simulink model "Quad_Nonlinear_Pitch_OL"  (R2020a)
settings: Solver=ode4  StartTime=0.0  StopTime=0.4  FixedStep=0.02  RelTol=1e-3
values from neighbouring files (symbols this model uses):
  B1 = (h_cg * g * m_tot) / (m_tot * h_cg^2 + J_yy)    [QuadConstants.m]    (also in pitch_parameter_estiation_result.m = 4.3602681386)
  B3 = (b * d_cg) / (m_tot * h_cg^2 + J_yy)    [QuadConstants.m]    (also in pitch_parameter_estiation_result.m = 7.12739951624e-05)
  B5 = (m2 * g * miu_k * r_y) / (m_tot * h_cg^2 + J_yy)    [QuadConstants.m]    (also in pitch_parameter_estiation_result.m = 0.59598011023)
  B6 = 2    [QuadConstants.m]    (also in pitch_parameter_estiation_result.m = 4.42876359313)
  init_I = data_I(1, :)    [load_data.m]
  init_II = data_II(1, :)    [load_data.m]
  init_III = data_III(1, :)    [load_data.m]
  init_IV = data_IV(1, :)    [load_data.m]
  init_V = data_V(1, :)    [load_data.m]
undefined symbols (not defined in the file or in its folder): magnitude
settings Model: OrderedModelArguments=off  Creator=Ali  LastModifiedBy=Ali

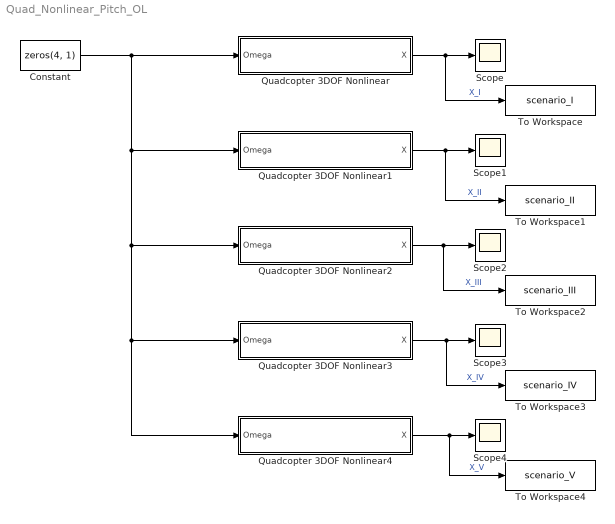
== system Quad_Nonlinear_Pitch_OL ==
  Constant : Constant  Value=zeros(4, 1)
  Quadcopter 3DOF Nonlinear : Subsystem  TreatAsAtomicUnit=on
  Quadcopter 3DOF Nonlinear1 : Subsystem  TreatAsAtomicUnit=on
  Quadcopter 3DOF Nonlinear2 : Subsystem  TreatAsAtomicUnit=on
  Quadcopter 3DOF Nonlinear3 : Subsystem  TreatAsAtomicUnit=on
  Quadcopter 3DOF Nonlinear4 : Subsystem  TreatAsAtomicUnit=on
  Scope{,1..4} (5 alike) : Scope
  To Workspace : ToWorkspace  VariableName=scenario_I  SampleTime=-1
  To Workspace1 : ToWorkspace  VariableName=scenario_II  SampleTime=-1
  To Workspace2 : ToWorkspace  VariableName=scenario_III  SampleTime=-1
  To Workspace3 : ToWorkspace  VariableName=scenario_IV  SampleTime=-1
  To Workspace4 : ToWorkspace  VariableName=scenario_V  SampleTime=-1
  wires:
  Quadcopter 3DOF Nonlinear/1(X) -> To Workspace/1, Scope/1  "X_I"
  Quadcopter 3DOF Nonlinear1/1(X) -> To Workspace1/1, Scope1/1  "X_II"
  Quadcopter 3DOF Nonlinear2/1(X) -> To Workspace2/1, Scope2/1  "X_III"
  Quadcopter 3DOF Nonlinear3/1(X) -> To Workspace3/1, Scope3/1  "X_IV"
  Quadcopter 3DOF Nonlinear4/1(X) -> To Workspace4/1, Scope4/1  "X_V"
  Constant/1 -> Quadcopter 3DOF Nonlinear4/1(Omega), Quadcopter 3DOF Nonlinear3/1(Omega), Quadcopter 3DOF Nonlinear2/1(Omega), Quadcopter 3DOF Nonlinear1/1(Omega), Quadcopter 3DOF Nonlinear/1(Omega)

== system Quad_Nonlinear_Pitch_OL/Quadcopter 3DOF Nonlinear ==
  Omega : Inport
  Integrator : Integrator  InitialCondition=init_I
  Quad System : Subsystem
  X : Outport
  wires:
  Integrator/1 -> Quad System/1(X), X/1  "X"
  Quad System/1(dot(X)) -> Integrator/1  "dot(X)"
  Omega/1 -> Quad System/2(Omega)

== system Quad_Nonlinear_Pitch_OL/Quadcopter 3DOF Nonlinear1 ==
  Omega : Inport
  Integrator : Integrator  InitialCondition=init_II
  Quad System : Subsystem
  X : Outport
  wires:
  Integrator/1 -> Quad System/1(X), X/1  "X"
  Quad System/1(dot(X)) -> Integrator/1  "dot(X)"
  Omega/1 -> Quad System/2(Omega)

== system Quad_Nonlinear_Pitch_OL/Quadcopter 3DOF Nonlinear2 ==
  Omega : Inport
  Integrator : Integrator  InitialCondition=init_III
  Quad System : Subsystem
  X : Outport
  wires:
  Integrator/1 -> Quad System/1(X), X/1  "X"
  Quad System/1(dot(X)) -> Integrator/1  "dot(X)"
  Omega/1 -> Quad System/2(Omega)

== system Quad_Nonlinear_Pitch_OL/Quadcopter 3DOF Nonlinear3 ==
  Omega : Inport
  Integrator : Integrator  InitialCondition=init_IV
  Quad System : Subsystem
  X : Outport
  wires:
  Integrator/1 -> Quad System/1(X), X/1  "X"
  Quad System/1(dot(X)) -> Integrator/1  "dot(X)"
  Omega/1 -> Quad System/2(Omega)

== system Quad_Nonlinear_Pitch_OL/Quadcopter 3DOF Nonlinear4 ==
  Omega : Inport
  Integrator : Integrator  InitialCondition=init_V
  Quad System : Subsystem
  X : Outport
  wires:
  Integrator/1 -> Quad System/1(X), X/1  "X"
  Quad System/1(dot(X)) -> Integrator/1  "dot(X)"
  Omega/1 -> Quad System/2(Omega)

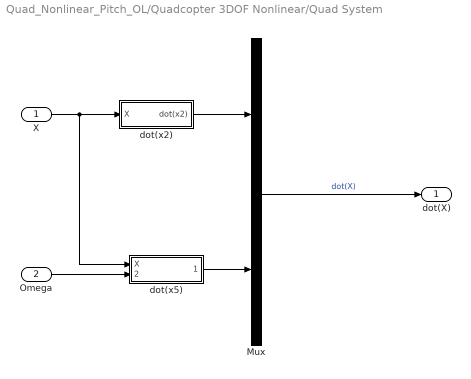
== system Quad_Nonlinear_Pitch_OL/Quadcopter 3DOF Nonlinear/Quad System ==
  X : Inport
  Omega : Inport  Port=2
  Mux : Mux  Inputs=2
  dot(x2) : Subsystem
  dot(x5) : Subsystem
  dot(X) : Outport
  wires:
  Mux/1 -> dot(X)/1  "dot(X)"
  dot(x2)/1(dot(x2)) -> Mux/1
  dot(x5)/1(dot(x5)) -> Mux/2
  X/1 -> dot(x5)/1(X), dot(x2)/1(X)
  Omega/1 -> dot(x5)/2(Omega)

== system Quad_Nonlinear_Pitch_OL/Quadcopter 3DOF Nonlinear1/Quad System ==
  X : Inport
  Omega : Inport  Port=2
  Mux : Mux  Inputs=2
  dot(x2) : Subsystem
  dot(x5) : Subsystem
  dot(X) : Outport
  wires:
  Mux/1 -> dot(X)/1  "dot(X)"
  dot(x2)/1(dot(x2)) -> Mux/1
  dot(x5)/1(dot(x5)) -> Mux/2
  X/1 -> dot(x5)/1(X), dot(x2)/1(X)
  Omega/1 -> dot(x5)/2(Omega)

== system Quad_Nonlinear_Pitch_OL/Quadcopter 3DOF Nonlinear2/Quad System ==
  X : Inport
  Omega : Inport  Port=2
  Mux : Mux  Inputs=2
  dot(x2) : Subsystem
  dot(x5) : Subsystem
  dot(X) : Outport
  wires:
  Mux/1 -> dot(X)/1  "dot(X)"
  dot(x2)/1(dot(x2)) -> Mux/1
  dot(x5)/1(dot(x5)) -> Mux/2
  X/1 -> dot(x5)/1(X), dot(x2)/1(X)
  Omega/1 -> dot(x5)/2(Omega)

== system Quad_Nonlinear_Pitch_OL/Quadcopter 3DOF Nonlinear3/Quad System ==
  X : Inport
  Omega : Inport  Port=2
  Mux : Mux  Inputs=2
  dot(x2) : Subsystem
  dot(x5) : Subsystem
  dot(X) : Outport
  wires:
  Mux/1 -> dot(X)/1  "dot(X)"
  dot(x2)/1(dot(x2)) -> Mux/1
  dot(x5)/1(dot(x5)) -> Mux/2
  X/1 -> dot(x5)/1(X), dot(x2)/1(X)
  Omega/1 -> dot(x5)/2(Omega)

== system Quad_Nonlinear_Pitch_OL/Quadcopter 3DOF Nonlinear4/Quad System ==
  X : Inport
  Omega : Inport  Port=2
  Mux : Mux  Inputs=2
  dot(x2) : Subsystem
  dot(x5) : Subsystem
  dot(X) : Outport
  wires:
  Mux/1 -> dot(X)/1  "dot(X)"
  dot(x2)/1(dot(x2)) -> Mux/1
  dot(x5)/1(dot(x5)) -> Mux/2
  X/1 -> dot(x5)/1(X), dot(x2)/1(X)
  Omega/1 -> dot(x5)/2(Omega)

== system Quad_Nonlinear_Pitch_OL/Quadcopter 3DOF Nonlinear/Quad System/dot(x2) ==
  X : Inport
  1 : Subsystem
  dot(x2) : Outport
  wires:
  X/1 -> 1/1(X)  "X"
  1/1(x5cos(x1)) -> dot(x2)/1

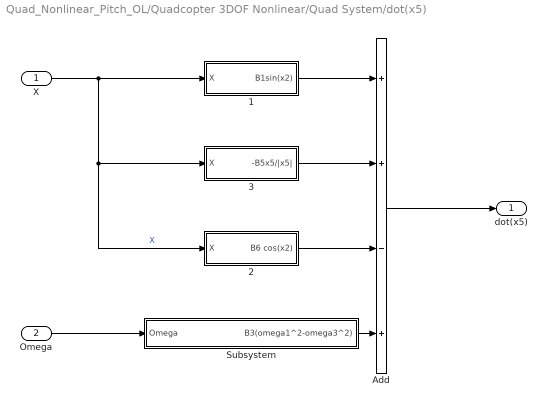
== system Quad_Nonlinear_Pitch_OL/Quadcopter 3DOF Nonlinear/Quad System/dot(x5) ==
  X : Inport
  Omega : Inport  Port=2
  1 : Subsystem
  2 : Subsystem
  3 : Subsystem
  Add : Sum  Inputs=++-+
  Subsystem : Subsystem
  dot(x5) : Outport
  wires:
  X/1 -> 2/1(X), 3/1(X), 1/1(X)  "X"
  Omega/1 -> Subsystem/1(Omega)
  Add/1 -> dot(x5)/1
  3/1("-B5x5/|x5| ") -> Add/2
  1/1(B1sin(x2)) -> Add/1
  Subsystem/1(B3(omega1^2-omega3^2)) -> Add/4
  2/1(B6 cos(x2)) -> Add/3

== system Quad_Nonlinear_Pitch_OL/Quadcopter 3DOF Nonlinear1/Quad System/dot(x2) ==
  X : Inport
  1 : Subsystem
  dot(x2) : Outport
  wires:
  X/1 -> 1/1(X)  "X"
  1/1(x5cos(x1)) -> dot(x2)/1

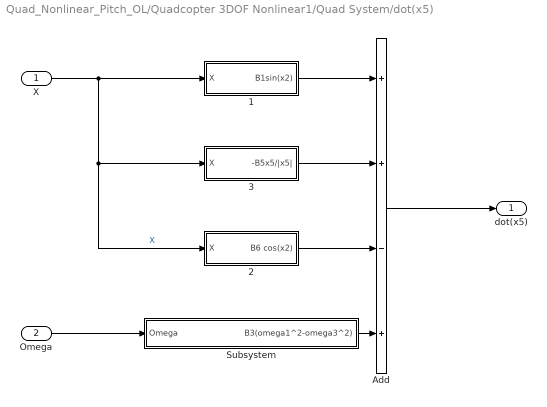
== system Quad_Nonlinear_Pitch_OL/Quadcopter 3DOF Nonlinear1/Quad System/dot(x5) ==
  X : Inport
  Omega : Inport  Port=2
  1 : Subsystem
  2 : Subsystem
  3 : Subsystem
  Add : Sum  Inputs=++-+
  Subsystem : Subsystem
  dot(x5) : Outport
  wires:
  X/1 -> 2/1(X), 3/1(X), 1/1(X)  "X"
  Omega/1 -> Subsystem/1(Omega)
  Add/1 -> dot(x5)/1
  3/1("-B5x5/|x5| ") -> Add/2
  1/1(B1sin(x2)) -> Add/1
  Subsystem/1(B3(omega1^2-omega3^2)) -> Add/4
  2/1(B6 cos(x2)) -> Add/3

== system Quad_Nonlinear_Pitch_OL/Quadcopter 3DOF Nonlinear2/Quad System/dot(x2) ==
  X : Inport
  1 : Subsystem
  dot(x2) : Outport
  wires:
  X/1 -> 1/1(X)  "X"
  1/1(x5cos(x1)) -> dot(x2)/1

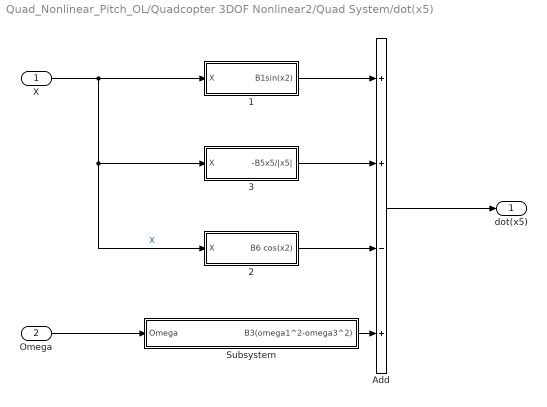
== system Quad_Nonlinear_Pitch_OL/Quadcopter 3DOF Nonlinear2/Quad System/dot(x5) ==
  X : Inport
  Omega : Inport  Port=2
  1 : Subsystem
  2 : Subsystem
  3 : Subsystem
  Add : Sum  Inputs=++-+
  Subsystem : Subsystem
  dot(x5) : Outport
  wires:
  X/1 -> 2/1(X), 3/1(X), 1/1(X)  "X"
  Omega/1 -> Subsystem/1(Omega)
  Add/1 -> dot(x5)/1
  3/1("-B5x5/|x5| ") -> Add/2
  1/1(B1sin(x2)) -> Add/1
  Subsystem/1(B3(omega1^2-omega3^2)) -> Add/4
  2/1(B6 cos(x2)) -> Add/3

== system Quad_Nonlinear_Pitch_OL/Quadcopter 3DOF Nonlinear3/Quad System/dot(x2) ==
  X : Inport
  1 : Subsystem
  dot(x2) : Outport
  wires:
  X/1 -> 1/1(X)  "X"
  1/1(x5cos(x1)) -> dot(x2)/1

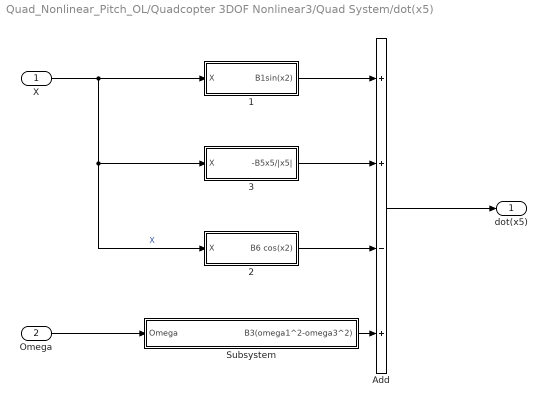
== system Quad_Nonlinear_Pitch_OL/Quadcopter 3DOF Nonlinear3/Quad System/dot(x5) ==
  X : Inport
  Omega : Inport  Port=2
  1 : Subsystem
  2 : Subsystem
  3 : Subsystem
  Add : Sum  Inputs=++-+
  Subsystem : Subsystem
  dot(x5) : Outport
  wires:
  X/1 -> 2/1(X), 3/1(X), 1/1(X)  "X"
  Omega/1 -> Subsystem/1(Omega)
  Add/1 -> dot(x5)/1
  3/1("-B5x5/|x5| ") -> Add/2
  1/1(B1sin(x2)) -> Add/1
  Subsystem/1(B3(omega1^2-omega3^2)) -> Add/4
  2/1(B6 cos(x2)) -> Add/3

== system Quad_Nonlinear_Pitch_OL/Quadcopter 3DOF Nonlinear4/Quad System/dot(x2) ==
  X : Inport
  1 : Subsystem
  dot(x2) : Outport
  wires:
  X/1 -> 1/1(X)  "X"
  1/1(x5cos(x1)) -> dot(x2)/1

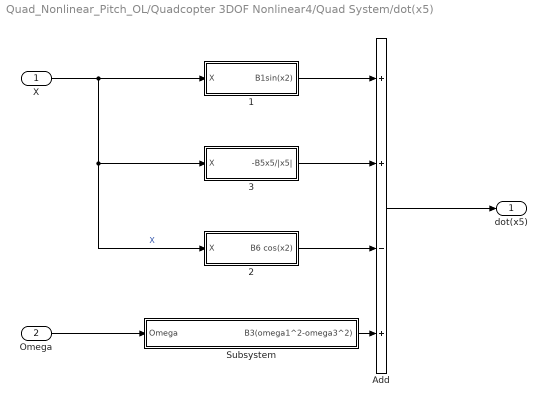
== system Quad_Nonlinear_Pitch_OL/Quadcopter 3DOF Nonlinear4/Quad System/dot(x5) ==
  X : Inport
  Omega : Inport  Port=2
  1 : Subsystem
  2 : Subsystem
  3 : Subsystem
  Add : Sum  Inputs=++-+
  Subsystem : Subsystem
  dot(x5) : Outport
  wires:
  X/1 -> 2/1(X), 3/1(X), 1/1(X)  "X"
  Omega/1 -> Subsystem/1(Omega)
  Add/1 -> dot(x5)/1
  3/1("-B5x5/|x5| ") -> Add/2
  1/1(B1sin(x2)) -> Add/1
  Subsystem/1(B3(omega1^2-omega3^2)) -> Add/4
  2/1(B6 cos(x2)) -> Add/3

== system Quad_Nonlinear_Pitch_OL/Quadcopter 3DOF Nonlinear/Quad System/dot(x2)/1 ==
  X : Inport
  Selector : Selector  InputPortWidth=2  IndexOptions=Index vector (dialog)  Indices=[2]  OutputSizes=1
  x5cos(x1) : Outport
  wires:
  X/1 -> Selector/1  "x"
  Selector/1 -> x5cos(x1)/1

== system Quad_Nonlinear_Pitch_OL/Quadcopter 3DOF Nonlinear/Quad System/dot(x5)/1 ==
  X : Inport
  Selector : Selector  InputPortWidth=2  IndexOptions=Index vector (dialog)  Indices=[1]  OutputSizes=1
  Subsystem : Subsystem
  B1sin(x2) : Outport
  wires:
  X/1 -> Selector/1  "x"
  Subsystem/1(B1sin(x2)) -> B1sin(x2)/1
  Selector/1 -> Subsystem/1(x2)

== system Quad_Nonlinear_Pitch_OL/Quadcopter 3DOF Nonlinear/Quad System/dot(x5)/2 ==
  X : Inport
  Selector : Selector  InputPortWidth=2  IndexOptions=Index vector (dialog)  Indices=[1]  OutputSizes=1
  Subsystem : Subsystem
  B6 cos(x2) : Outport
  wires:
  X/1 -> Selector/1  "x"
  Subsystem/1(B6 cos(x2)) -> B6 cos(x2)/1
  Selector/1 -> Subsystem/1(x2)

== system Quad_Nonlinear_Pitch_OL/Quadcopter 3DOF Nonlinear/Quad System/dot(x5)/3 ==
  X : Inport
  Selector : Selector  InputPortWidth=2  IndexOptions=Index vector (dialog)  Indices=[2]  OutputSizes=1
  Subsystem : Subsystem
  "-B5x5/|x5| " : Outport
  wires:
  X/1 -> Selector/1  "x"
  Subsystem/1("-B5x5/|x5| ") -> "-B5x5/|x5| "/1
  Selector/1 -> Subsystem/1(x5)

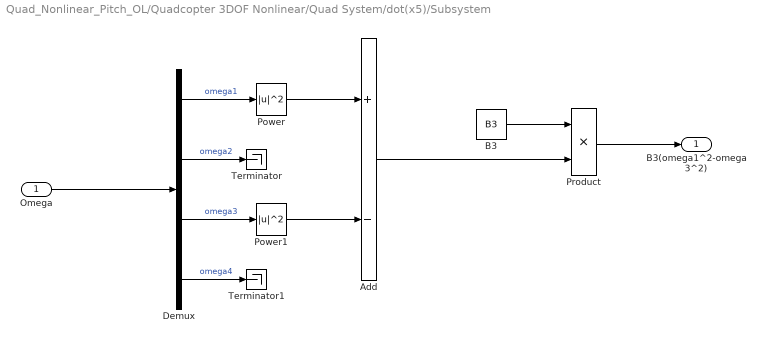
== system Quad_Nonlinear_Pitch_OL/Quadcopter 3DOF Nonlinear/Quad System/dot(x5)/Subsystem ==
  Omega : Inport
  Add : Sum  Inputs=+-
  B3 : Constant  Value=B3
  Demux : Demux
  Power : Math  Operator=magnitude^2  SaturateOnIntegerOverflow=on
  Power1 : Math  Operator=magnitude^2  SaturateOnIntegerOverflow=on
  Product : Product
  Terminator : Terminator
  Terminator1 : Terminator
  B3(omega1^2-omega3^2) : Outport
  wires:
  Product/1 -> B3(omega1^2-omega3^2)/1
  Power1/1 -> Add/2
  Add/1 -> Product/2
  Power/1 -> Add/1
  B3/1 -> Product/1
  Omega/1 -> Demux/1
  Demux/3 -> Power1/1  "omega3"
  Demux/1 -> Power/1  "omega1"
  Demux/2 -> Terminator/1  "omega2"
  Demux/4 -> Terminator1/1  "omega4"

== system Quad_Nonlinear_Pitch_OL/Quadcopter 3DOF Nonlinear1/Quad System/dot(x2)/1 ==
  X : Inport
  Selector : Selector  InputPortWidth=2  IndexOptions=Index vector (dialog)  Indices=[2]  OutputSizes=1
  x5cos(x1) : Outport
  wires:
  X/1 -> Selector/1  "x"
  Selector/1 -> x5cos(x1)/1

== system Quad_Nonlinear_Pitch_OL/Quadcopter 3DOF Nonlinear1/Quad System/dot(x5)/1 ==
  X : Inport
  Selector : Selector  InputPortWidth=2  IndexOptions=Index vector (dialog)  Indices=[1]  OutputSizes=1
  Subsystem : Subsystem
  B1sin(x2) : Outport
  wires:
  X/1 -> Selector/1  "x"
  Subsystem/1(B1sin(x2)) -> B1sin(x2)/1
  Selector/1 -> Subsystem/1(x2)

== system Quad_Nonlinear_Pitch_OL/Quadcopter 3DOF Nonlinear1/Quad System/dot(x5)/2 ==
  X : Inport
  Selector : Selector  InputPortWidth=2  IndexOptions=Index vector (dialog)  Indices=[1]  OutputSizes=1
  Subsystem : Subsystem
  B6 cos(x2) : Outport
  wires:
  X/1 -> Selector/1  "x"
  Subsystem/1(B6 cos(x2)) -> B6 cos(x2)/1
  Selector/1 -> Subsystem/1(x2)

== system Quad_Nonlinear_Pitch_OL/Quadcopter 3DOF Nonlinear1/Quad System/dot(x5)/3 ==
  X : Inport
  Selector : Selector  InputPortWidth=2  IndexOptions=Index vector (dialog)  Indices=[2]  OutputSizes=1
  Subsystem : Subsystem
  "-B5x5/|x5| " : Outport
  wires:
  X/1 -> Selector/1  "x"
  Subsystem/1("-B5x5/|x5| ") -> "-B5x5/|x5| "/1
  Selector/1 -> Subsystem/1(x5)

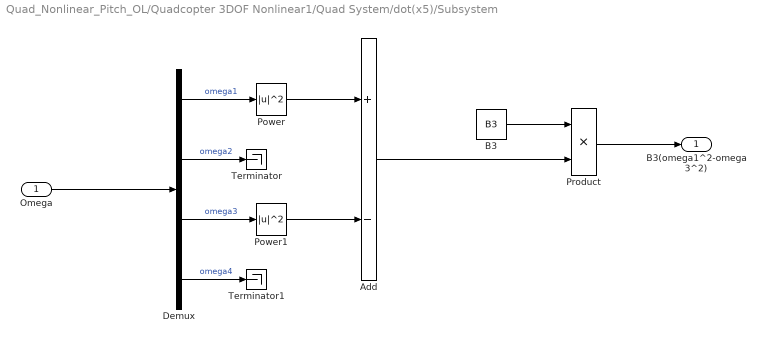
== system Quad_Nonlinear_Pitch_OL/Quadcopter 3DOF Nonlinear1/Quad System/dot(x5)/Subsystem ==
  Omega : Inport
  Add : Sum  Inputs=+-
  B3 : Constant  Value=B3
  Demux : Demux
  Power : Math  Operator=magnitude^2  SaturateOnIntegerOverflow=on
  Power1 : Math  Operator=magnitude^2  SaturateOnIntegerOverflow=on
  Product : Product
  Terminator : Terminator
  Terminator1 : Terminator
  B3(omega1^2-omega3^2) : Outport
  wires:
  Product/1 -> B3(omega1^2-omega3^2)/1
  Power1/1 -> Add/2
  Add/1 -> Product/2
  Power/1 -> Add/1
  B3/1 -> Product/1
  Omega/1 -> Demux/1
  Demux/3 -> Power1/1  "omega3"
  Demux/1 -> Power/1  "omega1"
  Demux/2 -> Terminator/1  "omega2"
  Demux/4 -> Terminator1/1  "omega4"

== system Quad_Nonlinear_Pitch_OL/Quadcopter 3DOF Nonlinear2/Quad System/dot(x2)/1 ==
  X : Inport
  Selector : Selector  InputPortWidth=2  IndexOptions=Index vector (dialog)  Indices=[2]  OutputSizes=1
  x5cos(x1) : Outport
  wires:
  X/1 -> Selector/1  "x"
  Selector/1 -> x5cos(x1)/1

== system Quad_Nonlinear_Pitch_OL/Quadcopter 3DOF Nonlinear2/Quad System/dot(x5)/1 ==
  X : Inport
  Selector : Selector  InputPortWidth=2  IndexOptions=Index vector (dialog)  Indices=[1]  OutputSizes=1
  Subsystem : Subsystem
  B1sin(x2) : Outport
  wires:
  X/1 -> Selector/1  "x"
  Subsystem/1(B1sin(x2)) -> B1sin(x2)/1
  Selector/1 -> Subsystem/1(x2)

== system Quad_Nonlinear_Pitch_OL/Quadcopter 3DOF Nonlinear2/Quad System/dot(x5)/2 ==
  X : Inport
  Selector : Selector  InputPortWidth=2  IndexOptions=Index vector (dialog)  Indices=[1]  OutputSizes=1
  Subsystem : Subsystem
  B6 cos(x2) : Outport
  wires:
  X/1 -> Selector/1  "x"
  Subsystem/1(B6 cos(x2)) -> B6 cos(x2)/1
  Selector/1 -> Subsystem/1(x2)

== system Quad_Nonlinear_Pitch_OL/Quadcopter 3DOF Nonlinear2/Quad System/dot(x5)/3 ==
  X : Inport
  Selector : Selector  InputPortWidth=2  IndexOptions=Index vector (dialog)  Indices=[2]  OutputSizes=1
  Subsystem : Subsystem
  "-B5x5/|x5| " : Outport
  wires:
  X/1 -> Selector/1  "x"
  Subsystem/1("-B5x5/|x5| ") -> "-B5x5/|x5| "/1
  Selector/1 -> Subsystem/1(x5)

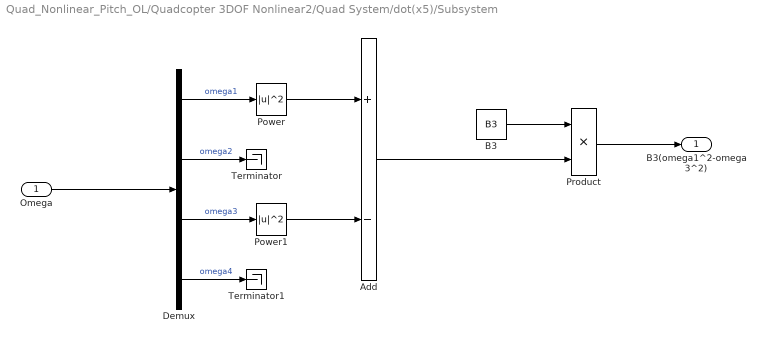
== system Quad_Nonlinear_Pitch_OL/Quadcopter 3DOF Nonlinear2/Quad System/dot(x5)/Subsystem ==
  Omega : Inport
  Add : Sum  Inputs=+-
  B3 : Constant  Value=B3
  Demux : Demux
  Power : Math  Operator=magnitude^2  SaturateOnIntegerOverflow=on
  Power1 : Math  Operator=magnitude^2  SaturateOnIntegerOverflow=on
  Product : Product
  Terminator : Terminator
  Terminator1 : Terminator
  B3(omega1^2-omega3^2) : Outport
  wires:
  Product/1 -> B3(omega1^2-omega3^2)/1
  Power1/1 -> Add/2
  Add/1 -> Product/2
  Power/1 -> Add/1
  B3/1 -> Product/1
  Omega/1 -> Demux/1
  Demux/3 -> Power1/1  "omega3"
  Demux/1 -> Power/1  "omega1"
  Demux/2 -> Terminator/1  "omega2"
  Demux/4 -> Terminator1/1  "omega4"

== system Quad_Nonlinear_Pitch_OL/Quadcopter 3DOF Nonlinear3/Quad System/dot(x2)/1 ==
  X : Inport
  Selector : Selector  InputPortWidth=2  IndexOptions=Index vector (dialog)  Indices=[2]  OutputSizes=1
  x5cos(x1) : Outport
  wires:
  X/1 -> Selector/1  "x"
  Selector/1 -> x5cos(x1)/1

== system Quad_Nonlinear_Pitch_OL/Quadcopter 3DOF Nonlinear3/Quad System/dot(x5)/1 ==
  X : Inport
  Selector : Selector  InputPortWidth=2  IndexOptions=Index vector (dialog)  Indices=[1]  OutputSizes=1
  Subsystem : Subsystem
  B1sin(x2) : Outport
  wires:
  X/1 -> Selector/1  "x"
  Subsystem/1(B1sin(x2)) -> B1sin(x2)/1
  Selector/1 -> Subsystem/1(x2)

== system Quad_Nonlinear_Pitch_OL/Quadcopter 3DOF Nonlinear3/Quad System/dot(x5)/2 ==
  X : Inport
  Selector : Selector  InputPortWidth=2  IndexOptions=Index vector (dialog)  Indices=[1]  OutputSizes=1
  Subsystem : Subsystem
  B6 cos(x2) : Outport
  wires:
  X/1 -> Selector/1  "x"
  Subsystem/1(B6 cos(x2)) -> B6 cos(x2)/1
  Selector/1 -> Subsystem/1(x2)

== system Quad_Nonlinear_Pitch_OL/Quadcopter 3DOF Nonlinear3/Quad System/dot(x5)/3 ==
  X : Inport
  Selector : Selector  InputPortWidth=2  IndexOptions=Index vector (dialog)  Indices=[2]  OutputSizes=1
  Subsystem : Subsystem
  "-B5x5/|x5| " : Outport
  wires:
  X/1 -> Selector/1  "x"
  Subsystem/1("-B5x5/|x5| ") -> "-B5x5/|x5| "/1
  Selector/1 -> Subsystem/1(x5)

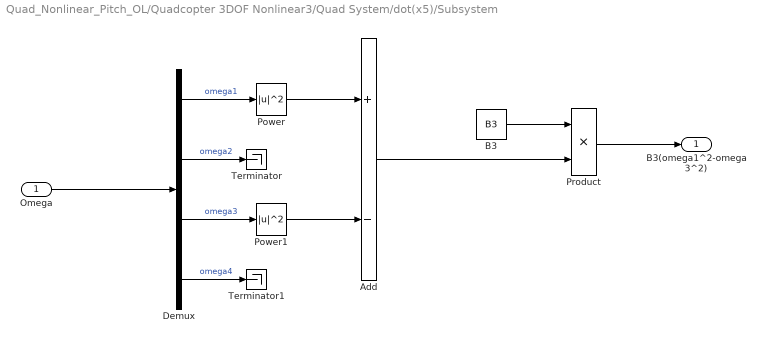
== system Quad_Nonlinear_Pitch_OL/Quadcopter 3DOF Nonlinear3/Quad System/dot(x5)/Subsystem ==
  Omega : Inport
  Add : Sum  Inputs=+-
  B3 : Constant  Value=B3
  Demux : Demux
  Power : Math  Operator=magnitude^2  SaturateOnIntegerOverflow=on
  Power1 : Math  Operator=magnitude^2  SaturateOnIntegerOverflow=on
  Product : Product
  Terminator : Terminator
  Terminator1 : Terminator
  B3(omega1^2-omega3^2) : Outport
  wires:
  Product/1 -> B3(omega1^2-omega3^2)/1
  Power1/1 -> Add/2
  Add/1 -> Product/2
  Power/1 -> Add/1
  B3/1 -> Product/1
  Omega/1 -> Demux/1
  Demux/3 -> Power1/1  "omega3"
  Demux/1 -> Power/1  "omega1"
  Demux/2 -> Terminator/1  "omega2"
  Demux/4 -> Terminator1/1  "omega4"

== system Quad_Nonlinear_Pitch_OL/Quadcopter 3DOF Nonlinear4/Quad System/dot(x2)/1 ==
  X : Inport
  Selector : Selector  InputPortWidth=2  IndexOptions=Index vector (dialog)  Indices=[2]  OutputSizes=1
  x5cos(x1) : Outport
  wires:
  X/1 -> Selector/1  "x"
  Selector/1 -> x5cos(x1)/1

== system Quad_Nonlinear_Pitch_OL/Quadcopter 3DOF Nonlinear4/Quad System/dot(x5)/1 ==
  X : Inport
  Selector : Selector  InputPortWidth=2  IndexOptions=Index vector (dialog)  Indices=[1]  OutputSizes=1
  Subsystem : Subsystem
  B1sin(x2) : Outport
  wires:
  X/1 -> Selector/1  "x"
  Subsystem/1(B1sin(x2)) -> B1sin(x2)/1
  Selector/1 -> Subsystem/1(x2)

== system Quad_Nonlinear_Pitch_OL/Quadcopter 3DOF Nonlinear4/Quad System/dot(x5)/2 ==
  X : Inport
  Selector : Selector  InputPortWidth=2  IndexOptions=Index vector (dialog)  Indices=[1]  OutputSizes=1
  Subsystem : Subsystem
  B6 cos(x2) : Outport
  wires:
  X/1 -> Selector/1  "x"
  Subsystem/1(B6 cos(x2)) -> B6 cos(x2)/1
  Selector/1 -> Subsystem/1(x2)

== system Quad_Nonlinear_Pitch_OL/Quadcopter 3DOF Nonlinear4/Quad System/dot(x5)/3 ==
  X : Inport
  Selector : Selector  InputPortWidth=2  IndexOptions=Index vector (dialog)  Indices=[2]  OutputSizes=1
  Subsystem : Subsystem
  "-B5x5/|x5| " : Outport
  wires:
  X/1 -> Selector/1  "x"
  Subsystem/1("-B5x5/|x5| ") -> "-B5x5/|x5| "/1
  Selector/1 -> Subsystem/1(x5)

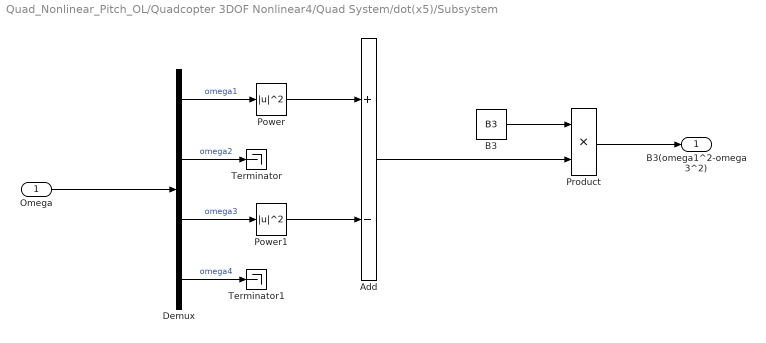
== system Quad_Nonlinear_Pitch_OL/Quadcopter 3DOF Nonlinear4/Quad System/dot(x5)/Subsystem ==
  Omega : Inport
  Add : Sum  Inputs=+-
  B3 : Constant  Value=B3
  Demux : Demux
  Power : Math  Operator=magnitude^2  SaturateOnIntegerOverflow=on
  Power1 : Math  Operator=magnitude^2  SaturateOnIntegerOverflow=on
  Product : Product
  Terminator : Terminator
  Terminator1 : Terminator
  B3(omega1^2-omega3^2) : Outport
  wires:
  Product/1 -> B3(omega1^2-omega3^2)/1
  Power1/1 -> Add/2
  Add/1 -> Product/2
  Power/1 -> Add/1
  B3/1 -> Product/1
  Omega/1 -> Demux/1
  Demux/3 -> Power1/1  "omega3"
  Demux/1 -> Power/1  "omega1"
  Demux/2 -> Terminator/1  "omega2"
  Demux/4 -> Terminator1/1  "omega4"

== system Quad_Nonlinear_Pitch_OL/Quadcopter 3DOF Nonlinear/Quad System/dot(x5)/1/Subsystem ==
  x2 : Inport
  B1 : Constant  Value=B1
  Product : Product
  Sin : Trigonometry
  B1sin(x2) : Outport
  wires:
  Product/1 -> B1sin(x2)/1
  x2/1 -> Sin/1
  B1/1 -> Product/2
  Sin/1 -> Product/1

== system Quad_Nonlinear_Pitch_OL/Quadcopter 3DOF Nonlinear/Quad System/dot(x5)/2/Subsystem ==
  x2 : Inport
  B6 : Constant  Value=B6
  Cos : Trigonometry  Operator=cos
  Product : Product
  B6 cos(x2) : Outport
  wires:
  B6/1 -> Product/1
  Product/1 -> B6 cos(x2)/1
  x2/1 -> Cos/1
  Cos/1 -> Product/2

== system Quad_Nonlinear_Pitch_OL/Quadcopter 3DOF Nonlinear/Quad System/dot(x5)/3/Subsystem ==
  x5 : Inport
  B5 : Constant  Value=B5
  Gain : Gain  Gain=-1
  Switch : Switch  Criteria=u2 > Threshold
  "-B5x5/|x5| " : Outport
  wires:
  Switch/1 -> "-B5x5/|x5| "/1
  B5/1 -> Switch/3, Gain/1
  x5/1 -> Switch/2
  Gain/1 -> Switch/1

== system Quad_Nonlinear_Pitch_OL/Quadcopter 3DOF Nonlinear1/Quad System/dot(x5)/1/Subsystem ==
  x2 : Inport
  B1 : Constant  Value=B1
  Product : Product
  Sin : Trigonometry
  B1sin(x2) : Outport
  wires:
  Product/1 -> B1sin(x2)/1
  x2/1 -> Sin/1
  B1/1 -> Product/2
  Sin/1 -> Product/1

== system Quad_Nonlinear_Pitch_OL/Quadcopter 3DOF Nonlinear1/Quad System/dot(x5)/2/Subsystem ==
  x2 : Inport
  B6 : Constant  Value=B6
  Cos : Trigonometry  Operator=cos
  Product : Product
  B6 cos(x2) : Outport
  wires:
  B6/1 -> Product/1
  Product/1 -> B6 cos(x2)/1
  x2/1 -> Cos/1
  Cos/1 -> Product/2

== system Quad_Nonlinear_Pitch_OL/Quadcopter 3DOF Nonlinear1/Quad System/dot(x5)/3/Subsystem ==
  x5 : Inport
  B5 : Constant  Value=B5
  Gain : Gain  Gain=-1
  Switch : Switch  Criteria=u2 > Threshold
  "-B5x5/|x5| " : Outport
  wires:
  Switch/1 -> "-B5x5/|x5| "/1
  B5/1 -> Switch/3, Gain/1
  x5/1 -> Switch/2
  Gain/1 -> Switch/1

== system Quad_Nonlinear_Pitch_OL/Quadcopter 3DOF Nonlinear2/Quad System/dot(x5)/1/Subsystem ==
  x2 : Inport
  B1 : Constant  Value=B1
  Product : Product
  Sin : Trigonometry
  B1sin(x2) : Outport
  wires:
  Product/1 -> B1sin(x2)/1
  x2/1 -> Sin/1
  B1/1 -> Product/2
  Sin/1 -> Product/1

== system Quad_Nonlinear_Pitch_OL/Quadcopter 3DOF Nonlinear2/Quad System/dot(x5)/2/Subsystem ==
  x2 : Inport
  B6 : Constant  Value=B6
  Cos : Trigonometry  Operator=cos
  Product : Product
  B6 cos(x2) : Outport
  wires:
  B6/1 -> Product/1
  Product/1 -> B6 cos(x2)/1
  x2/1 -> Cos/1
  Cos/1 -> Product/2

== system Quad_Nonlinear_Pitch_OL/Quadcopter 3DOF Nonlinear2/Quad System/dot(x5)/3/Subsystem ==
  x5 : Inport
  B5 : Constant  Value=B5
  Gain : Gain  Gain=-1
  Switch : Switch  Criteria=u2 > Threshold
  "-B5x5/|x5| " : Outport
  wires:
  Switch/1 -> "-B5x5/|x5| "/1
  B5/1 -> Switch/3, Gain/1
  x5/1 -> Switch/2
  Gain/1 -> Switch/1

== system Quad_Nonlinear_Pitch_OL/Quadcopter 3DOF Nonlinear3/Quad System/dot(x5)/1/Subsystem ==
  x2 : Inport
  B1 : Constant  Value=B1
  Product : Product
  Sin : Trigonometry
  B1sin(x2) : Outport
  wires:
  Product/1 -> B1sin(x2)/1
  x2/1 -> Sin/1
  B1/1 -> Product/2
  Sin/1 -> Product/1

== system Quad_Nonlinear_Pitch_OL/Quadcopter 3DOF Nonlinear3/Quad System/dot(x5)/2/Subsystem ==
  x2 : Inport
  B6 : Constant  Value=B6
  Cos : Trigonometry  Operator=cos
  Product : Product
  B6 cos(x2) : Outport
  wires:
  B6/1 -> Product/1
  Product/1 -> B6 cos(x2)/1
  x2/1 -> Cos/1
  Cos/1 -> Product/2

== system Quad_Nonlinear_Pitch_OL/Quadcopter 3DOF Nonlinear3/Quad System/dot(x5)/3/Subsystem ==
  x5 : Inport
  B5 : Constant  Value=B5
  Gain : Gain  Gain=-1
  Switch : Switch  Criteria=u2 > Threshold
  "-B5x5/|x5| " : Outport
  wires:
  Switch/1 -> "-B5x5/|x5| "/1
  B5/1 -> Switch/3, Gain/1
  x5/1 -> Switch/2
  Gain/1 -> Switch/1

== system Quad_Nonlinear_Pitch_OL/Quadcopter 3DOF Nonlinear4/Quad System/dot(x5)/1/Subsystem ==
  x2 : Inport
  B1 : Constant  Value=B1
  Product : Product
  Sin : Trigonometry
  B1sin(x2) : Outport
  wires:
  Product/1 -> B1sin(x2)/1
  x2/1 -> Sin/1
  B1/1 -> Product/2
  Sin/1 -> Product/1

== system Quad_Nonlinear_Pitch_OL/Quadcopter 3DOF Nonlinear4/Quad System/dot(x5)/2/Subsystem ==
  x2 : Inport
  B6 : Constant  Value=B6
  Cos : Trigonometry  Operator=cos
  Product : Product
  B6 cos(x2) : Outport
  wires:
  B6/1 -> Product/1
  Product/1 -> B6 cos(x2)/1
  x2/1 -> Cos/1
  Cos/1 -> Product/2

== system Quad_Nonlinear_Pitch_OL/Quadcopter 3DOF Nonlinear4/Quad System/dot(x5)/3/Subsystem ==
  x5 : Inport
  B5 : Constant  Value=B5
  Gain : Gain  Gain=-1
  Switch : Switch  Criteria=u2 > Threshold
  "-B5x5/|x5| " : Outport
  wires:
  Switch/1 -> "-B5x5/|x5| "/1
  B5/1 -> Switch/3, Gain/1
  x5/1 -> Switch/2
  Gain/1 -> Switch/1
